simulink model "position"  (R2022a)
settings: Solver=VariableStepAuto  StartTime=0.0  StopTime=10.0  RelTol=1e-3
settings Model: Creator=Lenovo  LastModifiedBy=Lenovo

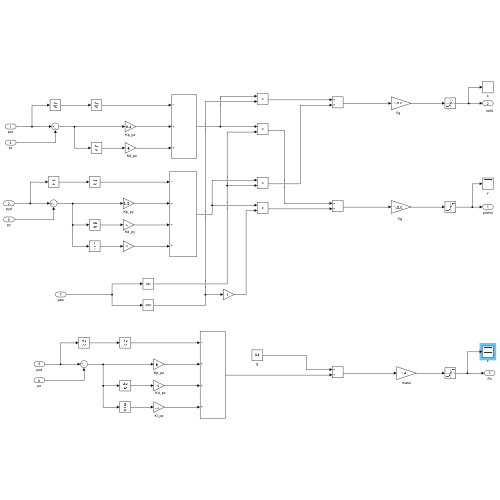
[thumbnail: Simulink's stored preview of the top-level diagram]
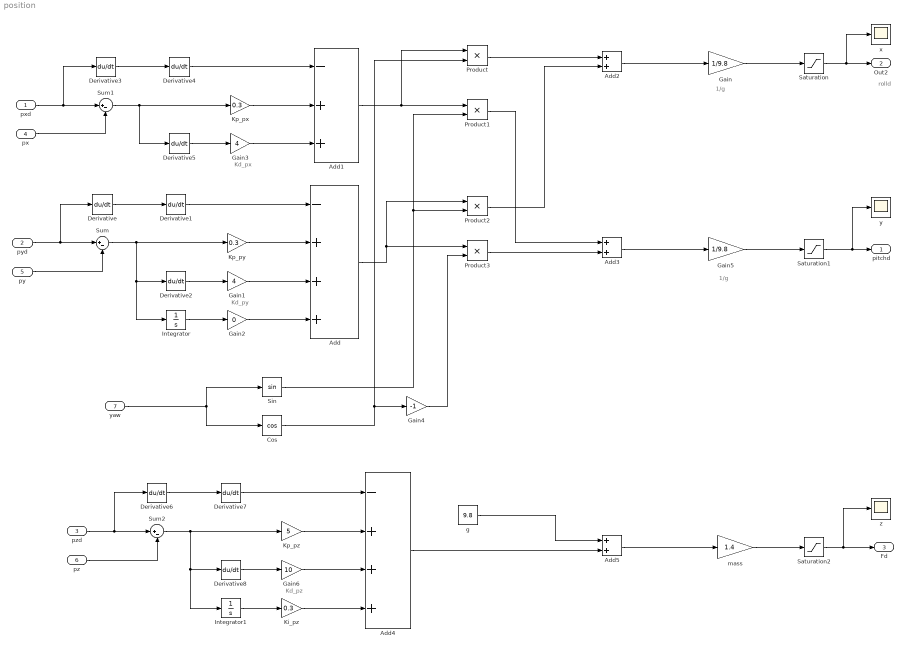
== system position ==
  note: rolld
  note: 1/g
  note: Kd_py
  note: Kd_px
  note: 1/g
  note: Kd_pz
  pxd : Inport
  pyd : Inport  Port=2
  pzd : Inport  Port=3
  px : Inport  Port=4
  py : Inport  Port=5
  pz : Inport  Port=6
  yaw : Inport  Port=7
  Add : Sum  Inputs=-+++
  Add1 : Sum  Inputs=-++
  Add2 : Sum
  Add3 : Sum
  Add4 : Sum  Inputs=-+++
  Add5 : Sum
  Cos : Trigonometry  Operator=cos
  Derivative{,1..8} (9 alike) : Derivative
  Gain : Gain  Gain=1/9.8
  Gain1 : Gain  Gain=4
  Gain2 : Gain  Gain=0
  Gain3 : Gain  Gain=4
  Gain4 : Gain  Gain=-1
  Gain5 : Gain  Gain=1/9.8
  Gain6 : Gain  Gain=10
  Integrator : Integrator
  Integrator1 : Integrator
  Ki_pz : Gain  Gain=0.3
  Kp_px : Gain  Gain=0.3
  Kp_py : Gain  Gain=0.3
  Kp_pz : Gain  Gain=5
  Product{,1..3} (4 alike) : Product
  Saturation : Saturate
  Saturation1 : Saturate
  Saturation2 : Saturate
  Sin : Trigonometry
  Sum : Sum  Inputs=|+-
  Sum1 : Sum  Inputs=|+-
  Sum2 : Sum  Inputs=|+-
  g : Constant  Value=9.8
  mass : Gain  Gain=1.4
  x : Scope
  y : Scope
  z : Scope
  pitchd : Outport
  Out2 : Outport  Port=2
  Fd : Outport  Port=3
  wires:
  Saturation2/1 -> Fd/1, z/1
  mass/1 -> Saturation2/1
  Add5/1 -> mass/1
  g/1 -> Add5/1
  Integrator1/1 -> Ki_pz/1
  Ki_pz/1 -> Add4/4
  Gain6/1 -> Add4/3
  Kp_pz/1 -> Add4/2
  Derivative7/1 -> Add4/1
  Derivative8/1 -> Gain6/1
  Sum2/1 -> Kp_pz/1, Derivative8/1, Integrator1/1
  Derivative6/1 -> Derivative7/1
  pz/1 -> Sum2/2
  pzd/1 -> Sum2/1, Derivative6/1
  Add4/1 -> Add5/2
  Saturation1/1 -> pitchd/1, y/1
  Saturation/1 -> Out2/1, x/1
  Gain5/1 -> Saturation1/1
  Gain/1 -> Saturation/1
  Add3/1 -> Gain5/1
  Add2/1 -> Gain/1
  Product3/1 -> Add3/2
  Product1/1 -> Add3/1
  Product2/1 -> Add2/2
  Product/1 -> Add2/1
  Add/1 -> Product3/1, Product2/1
  Gain4/1 -> Product3/2
  Cos/1 -> Product/2, Gain4/1
  Sin/1 -> Product1/2, Product2/2
  yaw/1 -> Sin/1, Cos/1
  Add1/1 -> Product1/1, Product/1
  pxd/1 -> Derivative3/1, Sum1/1
  px/1 -> Sum1/2
  Derivative3/1 -> Derivative4/1
  Sum1/1 -> Derivative5/1, Kp_px/1
  Derivative5/1 -> Gain3/1
  Derivative4/1 -> Add1/1
  Kp_px/1 -> Add1/2
  Gain3/1 -> Add1/3
  Gain2/1 -> Add/4
  Gain1/1 -> Add/3
  Kp_py/1 -> Add/2
  Derivative1/1 -> Add/1
  Derivative2/1 -> Gain1/1
  Integrator/1 -> Gain2/1
  Sum/1 -> Kp_py/1, Integrator/1, Derivative2/1
  Derivative/1 -> Derivative1/1
  py/1 -> Sum/2
  pyd/1 -> Sum/1, Derivative/1
